simulink model "FormulaElectric"  (R2015a)
settings: Solver=ode1  StartTime=0.0  StopTime=inf  FixedStep=0.001  RelTol=1e-3
InitFcn:
  | %init_dyn_platform
  | FEParameters
StartFcn:
  | tic
StopFcn:
  | toc
undefined symbols (not defined in the file): Battery, Env, magnitude, Motor, RPM2Rad
libraries: vehicleLib x22, mblibv1 x15, driveline x12, fl_lib x8, simulink x6, AMKMotor x4, nesl_utility x4, WheelAssembly x4, ephysenetlib x2, ControllerLib x1, simulink_extras x1
(part 4 of 4)

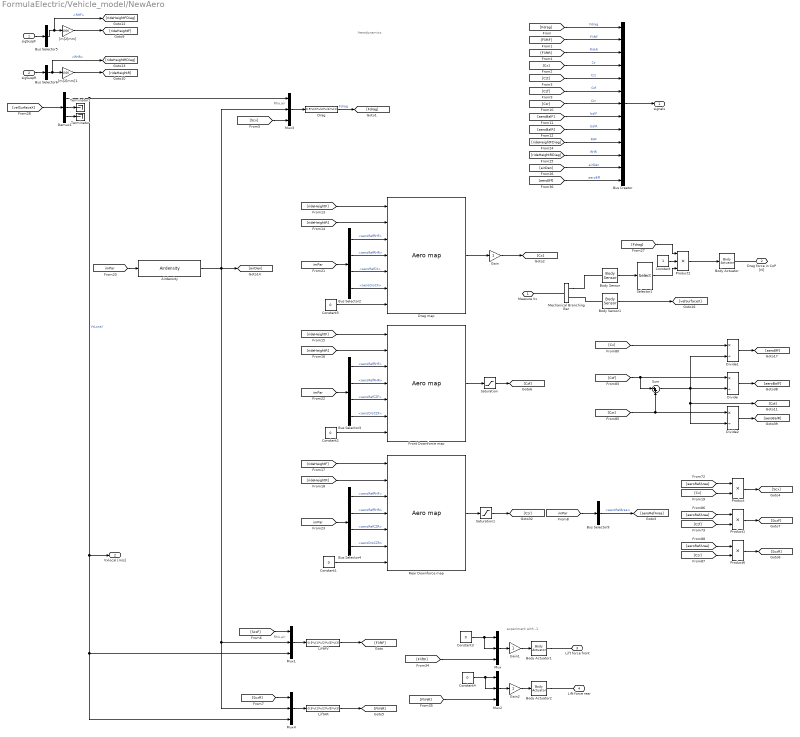
== system FormulaElectric/Vehicle_model/NewAero ==
  note: experiment with -1
  note: Rho,air
  note: Rho,air
  note: Aerodynamics
  sigSuspF : Inport
  sigSuspR : Inport  Port=2
  Airdensity : vehicleLib/Aerodynamics/Aero lib/Airdensity
  Body Actuator : mblibv1/Sensors &  Actuators/Body Actuator  UpdateFromCAD=off  PhysicalDomain=Mechanical  PortType=blob  ActuationStyle=Force  AngleUnits=deg  ArcVelocityUnits=deg/s  ArcAccelerationUnits=deg/s^2  CoordPositionUnits=m  VelocityUnits=m/s  AccelerationUnits=m/s^2  ForceUnits=N  TorqueUnits=N*m  ActiveIO=on  Width=3  DialogClass=MechanicalActuatorBlock  ReferenceFrame=Absolute (World)  Angle=off  CoordPosition=on  Force=on  Torque=off
  Body Actuator1 : mblibv1/Sensors &  Actuators/Body Actuator  UpdateFromCAD=off  PhysicalDomain=Mechanical  PortType=blob  ActuationStyle=Force  AngleUnits=deg  ArcVelocityUnits=deg/s  ArcAccelerationUnits=deg/s^2  CoordPositionUnits=m  VelocityUnits=m/s  AccelerationUnits=m/s^2  ForceUnits=N  TorqueUnits=N*m  ActiveIO=on  Width=3  DialogClass=MechanicalActuatorBlock  ReferenceFrame=Local (Body CS)  Angle=off  CoordPosition=on  Force=on  Torque=off
  Body Actuator2 : mblibv1/Sensors &  Actuators/Body Actuator  UpdateFromCAD=off  PhysicalDomain=Mechanical  PortType=blob  ActuationStyle=Force  AngleUnits=deg  ArcVelocityUnits=deg/s  ArcAccelerationUnits=deg/s^2  CoordPositionUnits=m  VelocityUnits=m/s  AccelerationUnits=m/s^2  ForceUnits=N  TorqueUnits=N*m  ActiveIO=on  Width=3  DialogClass=MechanicalActuatorBlock  ReferenceFrame=Local (Body CS)  Angle=off  CoordPosition=on  Force=on  Torque=off
  Body Sensor : mblibv1/Sensors &  Actuators/Body Sensor  UpdateFromCAD=off  PhysicalDomain=Mechanical  PortType=blob  Muxed=off  Pose=on  Angle=on  AngleUnits=deg  ArcVelocity=off  ArcVelocityUnits=deg/s  ArcAcceleration=off  ArcAccelerationUnits=deg/s^2  CoordPosition=off  CoordPositionUnits=m  Velocity=off  VelocityUnits=m/s  Acceleration=off  AccelerationUnits=m/s^2  Quaternion=on  QuaternionDT=off  QuaternionDDT=off  QuaternionUnits=off  OutputVector=[ 3 ]  ActiveIO=on  Width=9  DialogClass=MechanicalSensorBlock  ReferenceFrame=Absolute (World)
  Body Sensor1 : mblibv1/Sensors &  Actuators/Body Sensor  UpdateFromCAD=off  PhysicalDomain=Mechanical  PortType=blob  Muxed=off  Pose=off  Angle=on  AngleUnits=deg  ArcVelocity=off  ArcVelocityUnits=deg/s  ArcAcceleration=off  ArcAccelerationUnits=deg/s^2  CoordPosition=off  CoordPositionUnits=m  Velocity=on  VelocityUnits=m/s  Acceleration=off  AccelerationUnits=m/s^2  Quaternion=on  QuaternionDT=off  QuaternionDDT=off  QuaternionUnits=off  OutputVector=[ 3 ]  ActiveIO=on  Width=3  DialogClass=MechanicalSensorBlock  ReferenceFrame=Local (Body CS)
  Bus Creator : BusCreator  Inputs=13
  Bus Selector2 : BusSelector  OutputSignals=aeroRefRHF,aeroRefRHR,aeroRefCX,aeroDrsCX
  Bus Selector3 : BusSelector  OutputSignals=aeroRefRHF,aeroRefRHR,aeroRefCZF,aeroDrsCZF
  Bus Selector4 : BusSelector  OutputSignals=aeroRefRHF,aeroRefRHR,aeroRefCZR,aeroDrsCZR
  Bus Selector5 : BusSelector  OutputSignals=sigSuspRH.RHF
  Bus Selector6 : BusSelector  OutputSignals=sigSuspRH.RHR
  Bus Selector9 : BusSelector  OutputSignals=aeroRefArea
  Constant : Constant
  Constant{1..5} (5 alike) : Constant  Value=0
  Demux1 : Demux  Outputs=3
  Divide : Product  Inputs=*/
  Divide1 : Product  Inputs=*/
  Divide2 : Product  Inputs=*/
  Drag : Fcn  Expr=-0.5*u(2)*u(3)*u(1)*u(1)
  Drag map : vehicleLib/Aerodynamics/Aero lib/Aero map  Tag=Aerodynamics: aero map (do not change this tag)  nb=0
  Front Downforce map : vehicleLib/Aerodynamics/Aero lib/Aero map  Tag=Aerodynamics: aero map (do not change this tag)  nb=1
  Gain : Gain
  Gain1 : Gain
  Gain2 : Gain
  LiftAR : Fcn  Expr=-0.5*u(1)*u(2)*u(3)*u(3)
  LiftAV : Fcn  Expr=-0.5*u(1)*u(2)*u(3)*u(3)
  Mechanical Branching Bar : mblibv1/Utilities/Mechanical Branching Bar  LConnTagsString=_newl0  RConnTagsString=SA0|SA1  UpdateFromCAD=off  DialogClass=MechanicalBranchingBarBlock  NumSAPorts=2
  Mux{,1..4} (5 alike) : Mux  Inputs=3
  Product : Product  RndMeth=Zero
  Product1 : Product  RndMeth=Zero
  Product2 : Product  Inputs=3  RndMeth=Zero
  Product6 : Product  RndMeth=Zero
  Rear Downforce map : vehicleLib/Aerodynamics/Aero lib/Aero map  Tag=Aerodynamics: aero map (do not change this tag)  nb=2
  Saturation : Saturate  UpperLimit=0.2  LowerLimit=0
  Saturation1 : Saturate  UpperLimit=0.25  LowerLimit=0
  Selector1 : Selector  InputPortWidth=9  Indices=[1 2 3]
  Sum : Sum  Inputs=|++
  Terminator : Terminator
  Terminator1 : Terminator
  "[m]2[mm]" : Gain  Gain=1000
  "[m]2[mm]1" : Gain  Gain=1000
  Measure Vx : PMIOPort  Port=1  Side=Right
  Drag force in CoP [N] : PMIOPort  Port=2  Side=Left
  Lift force front : PMIOPort  Port=3  Side=Left
  Lift force rear : PMIOPort  Port=4  Side=Left
  signals : Outport
  Vxlocal [m/s] : Outport  Port=2
  wires:
  Constant/1 -> Product2/2
  Selector1/1 -> Product2/3
  Body Sensor/1 -> Selector1/1
  Product6/1 -> [SczR]
  [aeroRefArea] -> Product6/1
  [Czr] -> Product6/2
  Product1/1 -> [SczF]
  [aeroRefArea] -> Product1/1
  [Czf] -> Product1/2
  Product/1 -> [Scx]
  [aeroRefArea] -> Product/1
  [Cx] -> Product/2
  Bus Selector9/1 -> [aeroRefArea]  "<aeroRefArea>"
  [imPar] -> Bus Selector9/1
  Divide2/1 -> [aeroBalR]
  [Czr] -> Divide2/1, Sum/2
  Divide/1 -> [aeroBalF]
  [Czf] -> Divide/1, Sum/1
  Sum/1 -> Divide/2, [Czt], Divide2/2, Divide1/2
  [Cx] -> Divide1/1
  Bus Creator/1 -> signals/1
  [Fdrag] -> Bus Creator/1  "Fdrag"
  [FliftF] -> Bus Creator/2  "FliftF"
  [Cx] -> Bus Creator/4  "Cx"
  [Czt] -> Bus Creator/5  "Czt"
  [FliftR] -> Bus Creator/3  "FliftR"
  [aeroBalF] -> Bus Creator/8  "balF"
  [Czr] -> Bus Creator/7  "Czr"
  [Czf] -> Bus Creator/6  "Czf"
  [aeroBalR] -> Bus Creator/9  "balR"
  [rideHeightFDiag] -> Bus Creator/10  "RHF"
  [rideHeightRDiag] -> Bus Creator/11  "RHR"
  [airDen] -> Bus Creator/12  "airDen"
  [aeroEff] -> Bus Creator/13  "aeroEff"
  [FliftR] -> Mux2/3
  [FliftF] -> Mux/3
  LiftAV/1 -> [FliftF]
  Drag/1 -> [Fdrag]  "Fdrag"
  Mux1/1 -> LiftAV/1
  Mux3/1 -> Drag/1
  Airdensity/1 -> Mux3/2, Mux1/2, Mux4/2, [airDen]
  [Scx] -> Mux3/3
  [SczF] -> Mux1/1
  Mux4/1 -> LiftAR/1
  [SczR] -> Mux4/1
  LiftAR/1 -> [FliftR]
  "[m]2[mm]"/1 -> [rideHeightF]
  "[m]2[mm]1"/1 -> [rideHeightR]
  sigSuspF/1 -> Bus Selector5/1
  Bus Selector5/1 -> "[m]2[mm]"/1, [rideHeightFDiag]  "<RHF>"
  sigSuspR/1 -> Bus Selector6/1
  Bus Selector6/1 -> "[m]2[mm]1"/1, [rideHeightRDiag]  "<RHR>"
  Demux1/3 -> Terminator/1
  Demux1/2 -> Terminator1/1
  Demux1/1 -> Mux3/1, Mux1/3, Mux4/3, Vxlocal [m/s]/1  "VxLocal"
  [velSurfaceX] -> Demux1/1
  Mux/1 -> Gain1/1
  Mux2/1 -> Gain2/1
  Constant3/1 -> Mux/1, Mux/2
  Constant4/1 -> Mux2/1, Mux2/2
  [Fdrag] -> Product2/1
  Product2/1 -> Body Actuator/1
  Body Sensor1/1 -> [velSurfaceX]
  Drag map/1 -> Gain/1
  [rideHeightF] -> Drag map/1
  [imPar] -> Airdensity/1
  Divide1/1 -> [aeroEff]
  Bus Selector2/3 -> Drag map/5  "<aeroRefCX>"
  Bus Selector2/2 -> Drag map/4  "<aeroRefRHR>"
  Bus Selector2/4 -> Drag map/6  "<aeroDrsCX>"
  [imPar] -> Bus Selector2/1
  [rideHeightR] -> Drag map/2
  Bus Selector2/1 -> Drag map/3  "<aeroRefRHF>"
  Constant5/1 -> Drag map/7
  [rideHeightF] -> Front Downforce map/1
  [rideHeightR] -> Front Downforce map/2
  Constant2/1 -> Front Downforce map/7
  [rideHeightF] -> Rear Downforce map/1
  [rideHeightR] -> Rear Downforce map/2
  Constant1/1 -> Rear Downforce map/7
  Bus Selector3/1 -> Front Downforce map/3  "<aeroRefRHF>"
  [imPar] -> Bus Selector3/1
  Bus Selector3/4 -> Front Downforce map/6  "<aeroDrsCZF>"
  Bus Selector3/2 -> Front Downforce map/4  "<aeroRefRHR>"
  Bus Selector3/3 -> Front Downforce map/5  "<aeroRefCZF>"
  Bus Selector4/1 -> Rear Downforce map/3  "<aeroRefRHF>"
  [imPar] -> Bus Selector4/1
  Bus Selector4/4 -> Rear Downforce map/6  "<aeroDrsCZR>"
  Bus Selector4/2 -> Rear Downforce map/4  "<aeroRefRHR>"
  Bus Selector4/3 -> Rear Downforce map/5  "<aeroRefCZR>"
  Front Downforce map/1 -> Saturation/1
  Rear Downforce map/1 -> Saturation1/1
  Gain/1 -> [Cx]
  Saturation/1 -> [Czf]
  Saturation1/1 -> [Czr]
  Gain1/1 -> Body Actuator1/1
  Gain2/1 -> Body Actuator2/1
  connections:
  Body Sensor1/LConn1 -- Mechanical Branching Bar/RConn2
  Mechanical Branching Bar/RConn1 -- Body Sensor/LConn1
  Mechanical Branching Bar/LConn1 -- Measure Vx/RConn1
  Drag force in CoP [N]/RConn1 -- Body Actuator/RConn1
  Body Actuator1/RConn1 -- Lift force front/RConn1
  Body Actuator2/RConn1 -- Lift force rear/RConn1

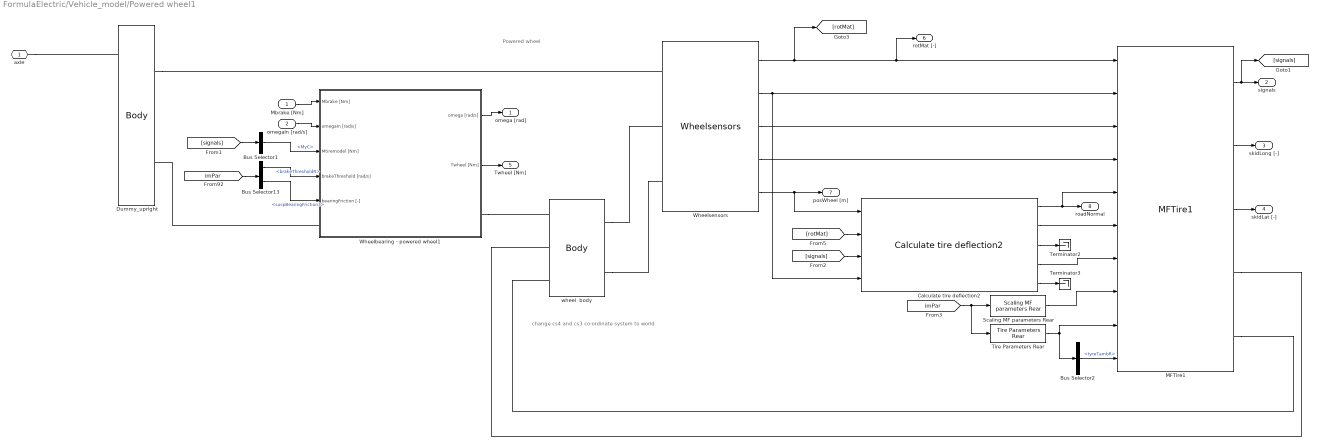
== system FormulaElectric/Vehicle_model/Powered wheel1 ==
  note: change cs4 and cs3 co-ordinate system to world
  note: Powered wheel
  Mbrake [Nm] : Inport
  omegaIn [rad/s] : Inport  Port=2
  Bus Selector1 : BusSelector  OutputSignals=MyC
  Bus Selector13 : BusSelector  OutputSignals=brakeThresholdR,suspBearingFriction3
  Bus Selector2 : BusSelector  OutputSignals=tyreTambR
  Calculate tire deflection2 : vehicleLib/Tire and rim/Tire lib/Calculate tire deflection2
  Dummy_upright : mblibv1/Bodies/Body  LConnTagsString=CS1|CS2|CS5  RConnTagsString=CS9|CS3  UpdateFromCAD=off  DialogClass=MechanicalBodyBlock  Mass=1e-3  MassUnits=kg  InertiaUnits=kg*m^2  Inertia=eye(3)*1e-6  Shape=Cylinder  ShapeDims=[1 1]  ShapeUnits=m  ShapeUse=false  Density=1  DensityUnits=kg/m^3  DensityUse=false  GraphicsMode=MACHINE_DEFAULT  BodyColorSelMode=MACHINE_DEFAULT  BodyColor=[1 0 0]  AttachedToCS=CG  CG=Left$CG$[0 0 0]$CS1$CS1$m$[0 0 0]$Euler X-Y-Z$deg$CS1$false$none  WorkingFrames=Left$CS1$[0 0 0]$Adjoining$Adjoining$m$[0 0 0]$Euler X-Y-Z$deg$Adjoining$true$none#Left$CS2$[suspX tw ahz]$World$World$m$[0 0 0]$Euler X-Y-Z$deg$WORLD$true$none#Right$CS9$[0 0 0]$CS2$CS2$m$[0 0 0]$Euler X-Y-Z$deg$WORLD$true$none#Right$CS3$[0 0 0]$CS1$CS1$m$[0 0 0]$Euler X-Y-Z$deg$CS1$true$none#Left$CS5$[0 0 0]$CS2$CS2$m$[0 0 0]$Euler X-Y-Z$deg$WORLD$true$none  CGPos=[0 0 0]  CGRot=[0 0 0]  CS0Pos=[]  CS0Rot=[]  CS1Pos=[0 0 0]  CS1Rot=[0 0 0]  CS2Pos=[suspX tw ahz]  CS2Rot=[0 0 0]  CS3Pos=[0 0 0]  CS3Rot=[0 0 0]  CS4Pos=[]  CS4Rot=[]  CS5Pos=[0 0 0]  CS5Rot=[0 0 0]  CS6Pos=[]  CS6Rot=[]  CS7Pos=[]  CS7Rot=[]  CS8Pos=[]  CS8Rot=[]  CS9Pos=[0 0 0]  CS9Rot=[0 0 0]  CS10Pos=[]  CS10Rot=[]  CS11Pos=[]  CS11Rot=[]  CS12Pos=[]  CS12Rot=[]  CS13Pos=[]  CS13Rot=[]  CS14Pos=[]  CS14Rot=[]  CS15Pos=[]  CS15Rot=[]  CS16Pos=[]  CS16Rot=[]  CS17Pos=[]  CS17Rot=[]  CS18Pos=[]  CS18Rot=[]  CS19Pos=[]  CS19Rot=[]  CS20Pos=[]  CS20Rot=[]
  MFTire1 : vehicleLib/Tire and rim/Tire lib/MFTire1
  Scaling MF parameters Rear : vehicleLib/Tire and rim/Tire lib/Scaling MF parameters Rear
  Terminator2 : Terminator
  Terminator3 : Terminator
  Tire Parameters Rear : vehicleLib/Tire and rim/Tire lib/Tire Parameters Rear
  Wheelbearing - powered wheel1 : Subsystem  Tag=Tire and rim: wheelbearing powered wheel (do not change this tag)  mask(Wheelbearing powered wheel){}
      mask help:
      | Wheelbearing powered wheel wheel model represents a wheelbearing with stick friction. To be used in combination with the SimMechanics multibody toolbox.
      |
      | Parameters in this model are only used for initialisation during the build process. During simulation with Racer Pro parameters are taken from the car.ini and/or relevant setup.ini.
      |
      | Wheelbearing powered wheel wheel model version: V1.0
      |
      | © Cruden B.V., 2012
  Wheelsensors : vehicleLib/Tire and rim/Tire lib/Wheelsensors
  wheel  body : mblibv1/Bodies/Body  LConnTagsString=CS1|CS2  RConnTagsString=CG|CS4|CS3  UpdateFromCAD=off  DialogClass=MechanicalBodyBlock  Mass=wheelMass  MassUnits=kg  InertiaUnits=kg*m^2  Inertia=inertiaWheel  Shape=Cylinder  ShapeDims=[1 1]  ShapeUnits=m  ShapeUse=false  Density=1  DensityUnits=kg/m^3  DensityUse=false  GraphicsMode=MACHINE_DEFAULT  BodyColorSelMode=MACHINE_DEFAULT  BodyColor=[1 0 0]  AttachedToCS=CG  CG=Right$CG$[0 0 0]$ADJOINING$ADJOINING$m$[0 0 0]$Euler X-Y-Z$deg$ADJOINING$true$none  WorkingFrames=Left$CS1$[0 0 0]$CG$CG$m$[0 0 0]$Euler X-Y-Z$deg$WORLD$true$none#Left$CS2$[0 0 0]$CG$CG$m$[0 0 0]$Euler X-Y-Z$deg$CG$true$none#Right$CS4$[0 0 0]$CG$CG$m$[0 0 0]$Euler X-Y-Z$deg$CG$true$none#Right$CS3$[0 0 0]$CG$CG$m$[0 0 0]$Euler X-Y-Z$deg$CG$true$none  CGPos=[0 0 0]  CGRot=[0 0 0]  CS0Pos=[]  CS0Rot=[]  CS1Pos=[0 0 0]  CS1Rot=[0 0 0]  CS2Pos=[0 0 0]  CS2Rot=[0 0 0]  CS3Pos=[0 0 0]  CS3Rot=[0 0 0]  CS4Pos=[0 0 0]  CS4Rot=[0 0 0]  CS5Pos=[]  CS5Rot=[]  CS6Pos=[]  CS6Rot=[]  CS7Pos=[]  CS7Rot=[]  CS8Pos=[]  CS8Rot=[]  CS9Pos=[]  CS9Rot=[]  CS10Pos=[]  CS10Rot=[]  CS11Pos=[]  CS11Rot=[]  CS12Pos=[]  CS12Rot=[]  CS13Pos=[]  CS13Rot=[]  CS14Pos=[]  CS14Rot=[]  CS15Pos=[]  CS15Rot=[]  CS16Pos=[]  CS16Rot=[]  CS17Pos=[]  CS17Rot=[]  CS18Pos=[]  CS18Rot=[]  CS19Pos=[]  CS19Rot=[]  CS20Pos=[]  CS20Rot=[]
  axle : PMIOPort  Port=1  Side=Left
  omega [rad] : Outport
  signals : Outport  Port=2
  skidLong [-] : Outport  Port=3
  skidLat [-] : Outport  Port=4
  Twheel [Nm] : Outport  Port=5
  rotMat [-] : Outport  Port=6
  posWheel [m] : Outport  Port=7
  roadNormal : Outport  Port=8
  wires:
  Wheelsensors/5 -> Calculate tire deflection2/1, posWheel [m]/1
  Calculate tire deflection2/2 -> MFTire1/6
  Calculate tire deflection2/4 -> MFTire1/7
  Scaling MF parameters Rear/1 -> MFTire1/8
  Bus Selector2/1 -> MFTire1/10  "<tyreTambR>"
  Calculate tire deflection2/5 -> Terminator3/1
  Calculate tire deflection2/3 -> Terminator2/1
  Wheelbearing - powered wheel1/1(omega [rad/s]) -> omega [rad]/1
  Bus Selector13/2 -> Wheelbearing - powered wheel1/5(bearingFriction [-])  "<suspBearingFriction3>"
  Bus Selector13/1 -> Wheelbearing - powered wheel1/4(brakeThreshold [rad/s])  "<brakeThresholdR>"
  [imPar] -> Bus Selector13/1
  Calculate tire deflection2/1 -> MFTire1/5, roadNormal/1
  [signals] -> Calculate tire deflection2/3
  [signals] -> Bus Selector1/1
  Wheelsensors/3 -> MFTire1/3
  Wheelsensors/2 -> Calculate tire deflection2/4, MFTire1/2
  Wheelsensors/1 -> rotMat [-]/1, MFTire1/1, [rotMat]
  MFTire1/1 -> signals/1, [signals]
  Tire Parameters Rear/1 -> MFTire1/9, Bus Selector2/1
  Wheelbearing - powered wheel1/2(Twheel [Nm]) -> Twheel [Nm]/1
  Mbrake [Nm]/1 -> Wheelbearing - powered wheel1/1(Mbrake [Nm])
  omegaIn [rad/s]/1 -> Wheelbearing - powered wheel1/2(omegaIn [rad/s])
  Bus Selector1/1 -> Wheelbearing - powered wheel1/3(Mtiremodel [Nm])  "<MyC>"
  [imPar] -> Scaling MF parameters Rear/1, Tire Parameters Rear/1
  [rotMat] -> Calculate tire deflection2/2
  MFTire1/2 -> skidLong [-]/1
  MFTire1/3 -> skidLat [-]/1
  Wheelsensors/4 -> MFTire1/4
  connections:
  Dummy_upright/RConn1 -- Wheelsensors/LConn1
  axle/RConn1 -- Dummy_upright/LConn1
  wheel  body/LConn1 -- Wheelsensors/LConn2
  wheel  body/LConn2 -- Wheelsensors/LConn3
  Wheelbearing - powered wheel1/RConn1 -- wheel  body/RConn1
  Wheelbearing - powered wheel1/LConn1 -- Dummy_upright/RConn2
  MFTire1/RConn2 -- wheel  body/RConn3
  MFTire1/RConn1 -- wheel  body/RConn2

== system FormulaElectric/Vehicle_model/Subsystem1 ==

== system FormulaElectric/Vehicle_model/World ==
  Custom Joint : mblibv1/Joints/Custom Joint  LConnTagsString=__newl0|SA1  RConnTagsString=__newr0  UpdateFromCAD=off  NumSAPorts=1  CutJoint=off  MarkAsCut=off  Primitives=prismatic  PrimitiveProps=P1$World$[1 0 0]$Prismatic#P2$World$[0 1 0]$Prismatic#P3$World$[0 0 1]$Prismatic#R1$World$[1 0 0]$revolute#R2$World$[0 1 0]$Revolute#R3$World$[0 0 1]$Revolute  DialogClass=JointBlock  R1Axis=[1 0 0]  R2Axis=[0 1 0]  R3Axis=[0 0 1]  P1Axis=[1 0 0]  P2Axis=[0 1 0]  P3Axis=[0 0 1]  SAxis=[]
  Ground : mblibv1/Bodies/Ground  UpdateFromCAD=off  LeftPortType=env  RightPortType=workingframe  PhysicalDomain=Mechanical  DialogClass=GroundBlock  CoordPosition=[0 0 0]  CoordPositionUnits=m  StateVectorMgrId=1  MachineId=[2 0]  ShowEnvPort=on  ParameterChecksum=[1644614091, 3398567388, 4103197596, 3842600041]  TopologyChecksum=[3388181360, 1225848865, 991958222, 3038121235]
  Joint Initial Condition : mblibv1/Sensors &  Actuators/Joint Initial Condition  UpdateFromCAD=off  LeftPortType=blob  RightPortType=blob  PhysicalDomain=mechanical  DialogClass=InitialConditionBlock  InitialConditions=P1$true$81.38$m$deg$0$m/s$deg/s#P2$true$2.75$m$deg$0$m/s$deg/s#P3$true$0$m$deg$0$m/s$deg/s#R1$false$0$m$deg$0$m/s$deg/s#R2$false$0$m$deg$0$m/s$deg/s#R3$false$0$m$deg$0$m/s$deg/s#S$false$0$m$deg$0$m/s$deg/s  P1PIC=81.38  P1VIC=0  P2PIC=2.75  P2VIC=0  P3PIC=0  P3VIC=0  R1PIC=0  R1VIC=0  R2PIC=0  R2VIC=0  R3PIC=0  R3VIC=0  SPIC=0  SVIC=0
  Machine Environment : mblibv1/Bodies/Machine Environment  Tag=Factory ground  PortType=env  PhysicalDomain=Mechanical  DialogTemplateClass=MECH.MachineEnvironment  SyncWhenCopied=off  Gravity=gravityVector  GravityUnits=m/s^2  GravityAsSignal=off  Dimensionality=3D Only  AnalysisType=Forward dynamics  LinearAssemblyTolerance=1e-3  LinearAssemblyToleranceUnits=m  AngularAssemblyTolerance=1e-3  AngularAssemblyToleranceUnits=rad  ConstraintSolverType=Stabilizing  ConstraintRelTolerance=1e-4  ConstraintAbsTolerance=1e-4  UseRobustSingularityHandling=off  RedundancyAnalysisToleranceType=Automatically select tolerance  RedundancyAnalysisTolerance=1e-14  StatePerturbationType=Fixed  PerturbationSize=1e-5  VisualizeMachine=on  BodyVisualizationType=Use model default body geometries  BodyColorSelMode=Use model default  DefaultBodyColor=[1 0 0]
  World : PMIOPort  Port=1  Side=Left
  connections:
  Custom Joint/RConn1 -- World/RConn1
  Custom Joint/LConn2 -- Joint Initial Condition/RConn1
  Machine Environment/RConn1 -- Ground/LConn1
  Custom Joint/LConn1 -- Ground/RConn1

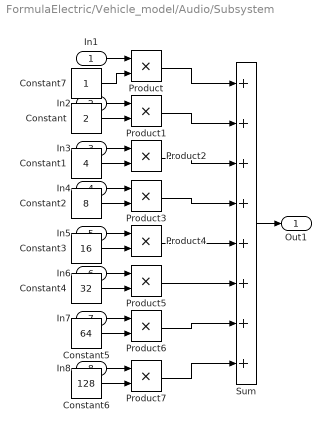
== system FormulaElectric/Vehicle_model/Audio/Subsystem ==
  In1 : Inport
  In2 : Inport  Port=2
  In3 : Inport  Port=3
  In4 : Inport  Port=4
  In5 : Inport  Port=5
  In6 : Inport  Port=6
  In7 : Inport  Port=7
  In8 : Inport  Port=8
  Constant : Constant  Value=2
  Constant1 : Constant  Value=4
  Constant2 : Constant  Value=8
  Constant3 : Constant  Value=16
  Constant4 : Constant  Value=32
  Constant5 : Constant  Value=64
  Constant6 : Constant  Value=128
  Constant7 : Constant
  Product{,1..7} (8 alike) : Product  RndMeth=Zero
  Sum : Sum  Inputs=++++++++
  Out1 : Outport
  wires:
  Constant7/1 -> Product/2
  Constant/1 -> Product1/2
  Constant1/1 -> Product2/2
  Constant2/1 -> Product3/2
  Constant3/1 -> Product4/2
  Constant4/1 -> Product5/2
  Constant5/1 -> Product6/2
  Constant6/1 -> Product7/2
  Product7/1 -> Sum/8
  Product6/1 -> Sum/7
  Product5/1 -> Sum/6
  Product4/1 -> Sum/5
  Product3/1 -> Sum/4
  Product2/1 -> Sum/3
  Product1/1 -> Sum/2
  Product/1 -> Sum/1
  In1/1 -> Product/1
  In2/1 -> Product1/1
  In3/1 -> Product2/1
  In4/1 -> Product3/1
  Sum/1 -> Out1/1
  In5/1 -> Product4/1
  In6/1 -> Product5/1
  In7/1 -> Product6/1
  In8/1 -> Product7/1

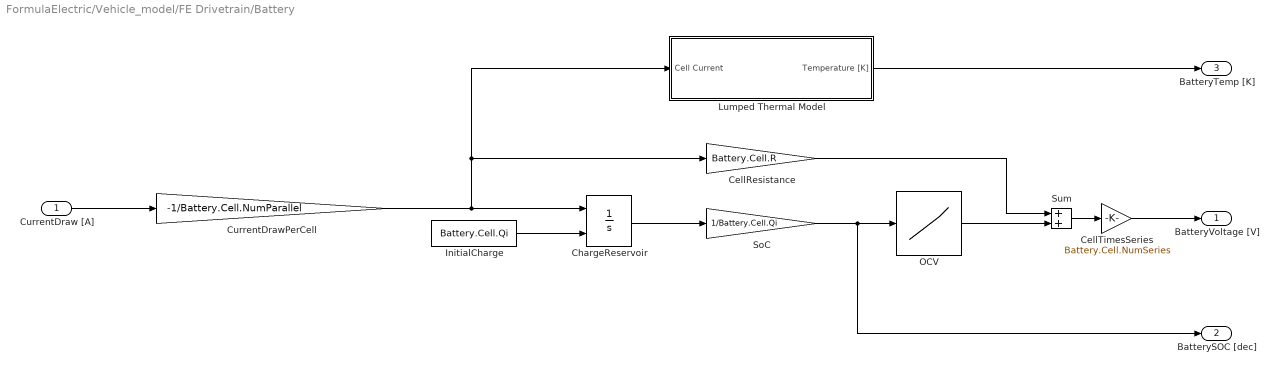
== system FormulaElectric/Vehicle_model/FE Drivetrain/Battery ==
  CurrentDraw [A] : Inport
  CellResistance : Gain  Gain=Battery.Cell.R
  CellTimesSeries : Gain  Gain=Battery.Cell.NumSeries
  ChargeReservoir : Integrator  InitialConditionSource=external
  CurrentDrawPerCell : Gain  Gain=-1/Battery.Cell.NumParallel
  InitialCharge : Constant  Value=Battery.Cell.Qi
  Lumped Thermal Model : Subsystem
  OCV : Lookup_n-D  NumberOfTableDimensions=1  BreakpointsForDimension1=Battery.Cell.VoltOC.SoC  Table=Battery.Cell.VoltOC.Voltage  InternalRulePriority=Speed  RndMeth=Simplest  InputSameDT=on
  SoC : Gain  Gain=1/Battery.Cell.Qi
  Sum : Sum
  BatteryVoltage [V] : Outport
  BatterySOC [dec] : Outport  Port=2
  BatteryTemp [K] : Outport  Port=3
  wires:
  Lumped Thermal Model/1(Temperature [K]) -> BatteryTemp [K]/1
  CurrentDrawPerCell/1 -> ChargeReservoir/1, CellResistance/1, Lumped Thermal Model/1(Cell Current)
  Sum/1 -> CellTimesSeries/1
  OCV/1 -> Sum/2
  CellResistance/1 -> Sum/1
  CellTimesSeries/1 -> BatteryVoltage [V]/1
  SoC/1 -> BatterySOC [dec]/1, OCV/1
  ChargeReservoir/1 -> SoC/1
  InitialCharge/1 -> ChargeReservoir/2
  CurrentDraw [A]/1 -> CurrentDrawPerCell/1

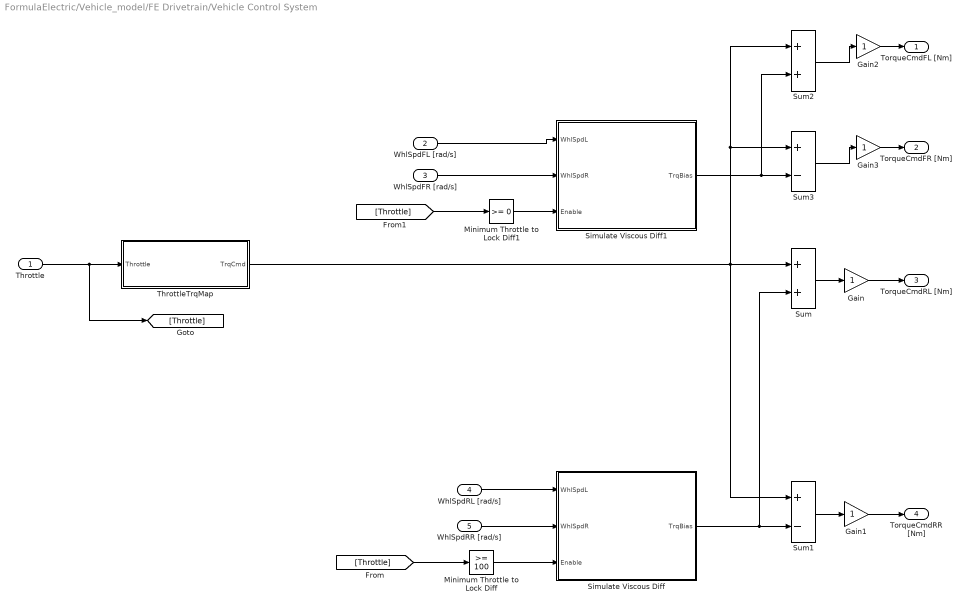
== system FormulaElectric/Vehicle_model/FE Drivetrain/Vehicle Control System ==
  Throttle : Inport
  WhlSpdFL [rad/s] : Inport  Port=2
  WhlSpdFR [rad/s] : Inport  Port=3
  WhlSpdRL [rad/s] : Inport  Port=4
  WhlSpdRR [rad/s] : Inport  Port=5
  Gain{,1..3} (4 alike) : Gain
  Minimum Throttle to Lock Diff : simulink/Logic and Bit Operations/Compare To Constant  relop=>=  const=100  OutDataTypeStr=boolean
  Minimum Throttle to Lock Diff1 : simulink/Logic and Bit Operations/Compare To Constant  relop=>=  const=0  OutDataTypeStr=boolean
  Simulate Viscous Diff : Subsystem
  Simulate Viscous Diff1 : Subsystem
  Sum : Sum
  Sum1 : Sum  Inputs=+-
  Sum2 : Sum
  Sum3 : Sum  Inputs=+-
  ThrottleTrqMap : Subsystem
  TorqueCmdFL [Nm] : Outport
  TorqueCmdFR [Nm] : Outport  Port=2
  TorqueCmdRL [Nm] : Outport  Port=3
  TorqueCmdRR [Nm] : Outport  Port=4
  wires:
  ThrottleTrqMap/1(TrqCmd) -> Sum3/1, Sum2/1, Sum1/1, Sum/1
  WhlSpdRL [rad/s]/1 -> Simulate Viscous Diff/1(WhlSpdL)
  WhlSpdRR [rad/s]/1 -> Simulate Viscous Diff/2(WhlSpdR)
  Simulate Viscous Diff/1(TrqBias) -> Sum1/2, Sum/2
  Sum/1 -> Gain/1
  Sum1/1 -> Gain1/1
  Throttle/1 -> [Throttle], ThrottleTrqMap/1(Throttle)
  [Throttle] -> Minimum Throttle to Lock Diff/1
  Minimum Throttle to Lock Diff/1 -> Simulate Viscous Diff/3(Enable)
  Gain/1 -> TorqueCmdRL [Nm]/1
  Gain1/1 -> TorqueCmdRR [Nm]/1
  WhlSpdFL [rad/s]/1 -> Simulate Viscous Diff1/1(WhlSpdL)
  WhlSpdFR [rad/s]/1 -> Simulate Viscous Diff1/2(WhlSpdR)
  [Throttle] -> Minimum Throttle to Lock Diff1/1
  Minimum Throttle to Lock Diff1/1 -> Simulate Viscous Diff1/3(Enable)
  Simulate Viscous Diff1/1(TrqBias) -> Sum2/2, Sum3/2
  Sum2/1 -> Gain2/1
  Sum3/1 -> Gain3/1
  Gain2/1 -> TorqueCmdFL [Nm]/1
  Gain3/1 -> TorqueCmdFR [Nm]/1

== system FormulaElectric/Vehicle_model/FE Drivetrain/Wheel Assembly ==
  WhlFdbkTrq [Nm] : Inport
  Motion Sensor1 : driveline/Sensors & Actuators/Motion Sensor  Angle=off  x0=0  Velocity=on  Acceleration=off
  Torque Actuator1 : driveline/Sensors & Actuators/Torque Actuator
  driveAxleInertiaR : driveline/Solver & Inertias/Inertia  PortType=p1  BlockClass=Inertia  PhysicalDomain=driveline_domain  I=0.5  Ip=[]  Iv=[]  ShowLeft=on  ShowRight=off
  WhlIn : PMIOPort  Port=1  Side=Left
  WheelSpeed [Rad/s] : Outport
  wires:
  Motion Sensor1/1 -> WheelSpeed [Rad/s]/1  "omegaR"
  WhlFdbkTrq [Nm]/1 -> Torque Actuator1/1
  connections:
  WhlIn/RConn1 -- Motion Sensor1/LConn1 -- Torque Actuator1/RConn1 -- driveAxleInertiaR/LConn1

== system FormulaElectric/Vehicle_model/FE Drivetrain/Wheel Assembly1 ==
  WhlFdbkTrq [Nm] : Inport
  Motion Sensor1 : driveline/Sensors & Actuators/Motion Sensor  Angle=off  x0=0  Velocity=on  Acceleration=off
  Torque Actuator1 : driveline/Sensors & Actuators/Torque Actuator
  driveAxleInertiaR : driveline/Solver & Inertias/Inertia  PortType=p1  BlockClass=Inertia  PhysicalDomain=driveline_domain  I=0.5  Ip=[]  Iv=[]  ShowLeft=on  ShowRight=off
  WhlIn : PMIOPort  Port=1  Side=Left
  WheelSpeed [Rad/s] : Outport
  wires:
  Motion Sensor1/1 -> WheelSpeed [Rad/s]/1  "omegaR"
  WhlFdbkTrq [Nm]/1 -> Torque Actuator1/1
  connections:
  WhlIn/RConn1 -- Motion Sensor1/LConn1 -- Torque Actuator1/RConn1 -- driveAxleInertiaR/LConn1

== system FormulaElectric/Vehicle_model/FE Drivetrain/Wheel Assembly2 ==
  WhlFdbkTrq [Nm] : Inport
  Motion Sensor1 : driveline/Sensors & Actuators/Motion Sensor  Angle=off  x0=0  Velocity=on  Acceleration=off
  Torque Actuator1 : driveline/Sensors & Actuators/Torque Actuator
  driveAxleInertiaR : driveline/Solver & Inertias/Inertia  PortType=p1  BlockClass=Inertia  PhysicalDomain=driveline_domain  I=0.5  Ip=[]  Iv=[]  ShowLeft=on  ShowRight=off
  WhlIn : PMIOPort  Port=1  Side=Left
  WheelSpeed [Rad/s] : Outport
  wires:
  Motion Sensor1/1 -> WheelSpeed [Rad/s]/1  "omegaR"
  WhlFdbkTrq [Nm]/1 -> Torque Actuator1/1
  connections:
  WhlIn/RConn1 -- Motion Sensor1/LConn1 -- Torque Actuator1/RConn1 -- driveAxleInertiaR/LConn1

== system FormulaElectric/Vehicle_model/FE Drivetrain/Wheel Assembly3 ==
  WhlFdbkTrq [Nm] : Inport
  Motion Sensor1 : driveline/Sensors & Actuators/Motion Sensor  Angle=off  x0=0  Velocity=on  Acceleration=off
  Torque Actuator1 : driveline/Sensors & Actuators/Torque Actuator
  driveAxleInertiaR : driveline/Solver & Inertias/Inertia  PortType=p1  BlockClass=Inertia  PhysicalDomain=driveline_domain  I=0.5  Ip=[]  Iv=[]  ShowLeft=on  ShowRight=off
  WhlIn : PMIOPort  Port=1  Side=Left
  WheelSpeed [Rad/s] : Outport
  wires:
  Motion Sensor1/1 -> WheelSpeed [Rad/s]/1  "omegaR"
  WhlFdbkTrq [Nm]/1 -> Torque Actuator1/1
  connections:
  WhlIn/RConn1 -- Motion Sensor1/LConn1 -- Torque Actuator1/RConn1 -- driveAxleInertiaR/LConn1

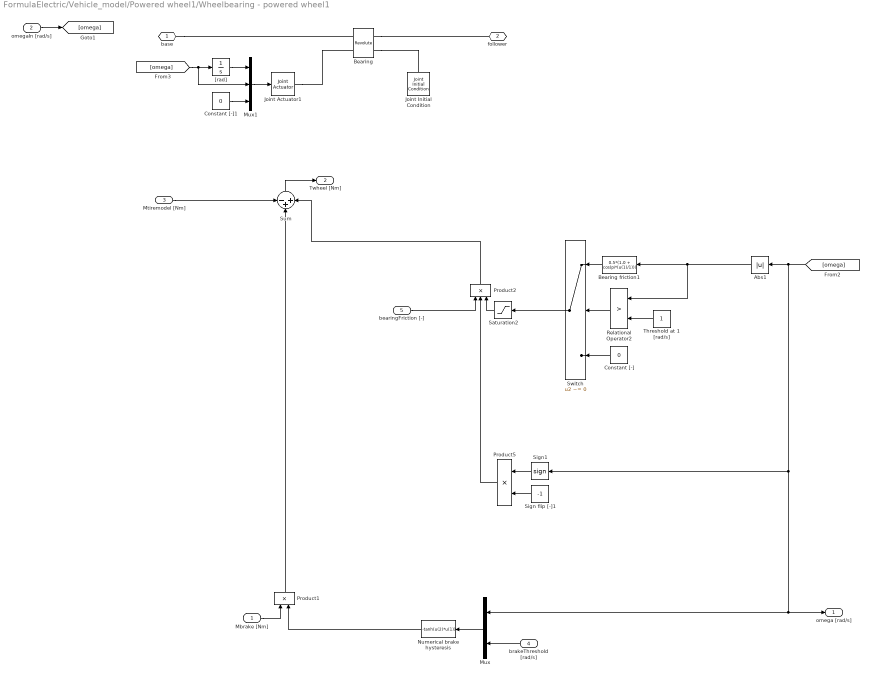
== system FormulaElectric/Vehicle_model/Powered wheel1/Wheelbearing - powered wheel1 ==
  Mbrake [Nm] : Inport
  omegaIn [rad/s] : Inport  Port=2
  Mtiremodel [Nm] : Inport  Port=3
  brakeThreshold [rad/s] : Inport  Port=4
  bearingFriction [-] : Inport  Port=5
  Abs1 : Abs
  Bearing : mblibv1/Joints/Revolute  LConnTagsString=__newl0|SA1  RConnTagsString=__newr0|SA1  UpdateFromCAD=off  NumSAPorts=2  CutJoint=off  MarkAsCut=off  Primitives=revolute  PrimitiveProps=R1$Base$[0 1 0]$revolute  DialogClass=JointBlock  R1Axis=[0 1 0]
  Bearing friction1 : Fcn  Expr=0.5*(1.0 + cos(pi*(u(1)/1)))
  Constant [-] : Constant  Value=0
  Constant [-]1 : Constant  Value=0
  Joint Actuator1 : mblibv1/Sensors &  Actuators/Joint Actuator  UpdateFromCAD=off  PhysicalDomain=Mechanical  PortType=blob  ActuationStyle=Motion  AngleUnits=rad  ArcVelocityUnits=rad/s  ArcAccelerationUnits=rad/s^2  CoordPositionUnits=m  VelocityUnits=m/s  AccelerationUnits=m/s^2  ForceUnits=N  TorqueUnits=N*m  ActiveIO=on  Width=3  DialogClass=MechanicalActuatorBlock  Primitive=R1  ReferenceFrame=Absolute (World)
  Joint Initial Condition : mblibv1/Sensors &  Actuators/Joint Initial Condition  UpdateFromCAD=off  LeftPortType=blob  RightPortType=blob  PhysicalDomain=Mechanical  DialogClass=InitialConditionBlock  InitialConditions=P1$false$0$m$rad$0$m/s$rad/s#P2$false$0$m$rad$0$m/s$rad/s#P3$false$0$m$rad$0$m/s$rad/s#R1$true$0$m$rad$0$m/s$rad/s#R2$false$0$m$rad$Vx/0.284$m/s$rad/s#R3$false$0$m$rad$0$m/s$rad/s#S$false$0$m$rad$0$m/s$rad/s  P1PIC=0  P1VIC=0  P2PIC=0  P2VIC=0  P3PIC=0  P3VIC=0  R1PIC=0  R1VIC=0  R2PIC=0  R2VIC=0  R3PIC=0  R3VIC=0  SPIC=0  SVIC=0
  Mux : Mux  Inputs=2
  Mux1 : Mux  Inputs=3
  Numerical brake hysteresis : Fcn  Expr=-tanh(u(2)*u(1))
  Product1 : Product  SaturateOnIntegerOverflow=on  InputSameDT=on  OutDataTypeStr=Inherit: Same as first input
  Product2 : Product  Inputs=3  SaturateOnIntegerOverflow=on  InputSameDT=on  OutDataTypeStr=Inherit: Same as first input
  Product5 : Product  SaturateOnIntegerOverflow=on  InputSameDT=on  OutDataTypeStr=Inherit: Same as first input
  Relational Operator2 : RelationalOperator  Operator=>  OutDataTypeStr=boolean
  Saturation2 : Saturate  UpperLimit=1  LowerLimit=0
  Sign flip [-]1 : Constant  Value=-1
  Sign1 : Signum
  Sum : Sum  Inputs=-++
  Switch : Switch  Criteria=u2 ~= 0
  Threshold at 1 [rad/s] : Constant
  "[rad]" : Integrator
  base : PMIOPort  Port=1  Side=Left
  follower : PMIOPort  Port=2  Side=Right
  omega [rad/s] : Outport
  Twheel [Nm] : Outport  Port=2
  wires:
  brakeThreshold [rad/s]/1 -> Mux/2
  Product2/1 -> Sum/3
  Sign flip [-]1/1 -> Product5/2
  bearingFriction [-]/1 -> Product2/1
  Switch/1 -> Saturation2/1
  Constant [-]/1 -> Switch/3
  Bearing friction1/1 -> Switch/1
  Relational Operator2/1 -> Switch/2
  Abs1/1 -> Bearing friction1/1, Relational Operator2/1
  Threshold at 1 [rad/s]/1 -> Relational Operator2/2
  [omega] -> Mux/1, omega [rad/s]/1, Sign1/1, Abs1/1
  Saturation2/1 -> Product2/3
  Sign1/1 -> Product5/1
  Product5/1 -> Product2/2
  [omega] -> Mux1/2, "[rad]"/1
  "[rad]"/1 -> Mux1/1
  Mux1/1 -> Joint Actuator1/1
  omegaIn [rad/s]/1 -> [omega]
  Product1/1 -> Sum/2
  Mtiremodel [Nm]/1 -> Sum/1
  Numerical brake hysteresis/1 -> Product1/2
  Mux/1 -> Numerical brake hysteresis/1
  Mbrake [Nm]/1 -> Product1/1
  Sum/1 -> Twheel [Nm]/1
  Constant [-]1/1 -> Mux1/3
  connections:
  Joint Actuator1/RConn1 -- Bearing/LConn2
  Bearing/RConn2 -- Joint Initial Condition/RConn1
  Bearing/RConn1 -- follower/RConn1
  base/RConn1 -- Bearing/LConn1

== system FormulaElectric/Vehicle_model/FE Drivetrain/Battery/Lumped Thermal Model ==
  Cell Current : Inport
  CellResistance1 : Gain  Gain=Battery.Cell.R
  Environment Air : Subsystem
  Heat Source : Subsystem
  Math Function : Math  Operator=magnitude^2  SaturateOnIntegerOverflow=on
  No_Cells : Gain  Gain=Battery.Cell.NumParallel * Battery.Cell.NumSeries
  Solver Configuration : nesl_utility/Solver Configuration  PhysicalDomain=network_engine_domain  SubClassName=solver  LeftPortType=input  RightPortType=generic  Accelerate=off  Tones=[]  Harmonics=[]  SimulateNoise=off  Profile=off  UseLocalSampling=off  EnableSwitchedLinearOptims=on  FrequencyDomain=off  UseCCode=off  RelTol=0.001  AbsTol=1e-06  MinStep=1e-09  ToWorkspace=off  RevertToSquareIcSolve=off  NumHomotopyIterations=100  DoDC=off  ResidualTolerance=1e-09  UseLocalSolver=off  LocalSolverChoice=NE_BACKWARD_EULER_ADVANCER  LocalSolverSampleTime=0.001  DoFixedCost=off  MaxNonlinIter=3  MaxModeIter=2  LinearAlgebra=Sparse  DelaysMemoryBudget=1024  AutomaticFiltering=on  FilteringTimeConstant=0.001
  Temperature Sensor : Subsystem
  Thermal Mass : fl_lib/Thermal/Thermal Elements/Thermal Mass  mass=Battery.m kg  sp_heat=Battery.c J/kg/K  Q_specify=off  Q_priority=High  Q=0 J/s  T_specify=off  T_priority=High  T=300 K
  Temperature [K] : Outport
  wires:
  Cell Current/1 -> Math Function/1
  Temperature Sensor/1(Temperature [K]) -> Temperature [K]/1
  No_Cells/1 -> Heat Source/1(Q)
  CellResistance1/1 -> No_Cells/1
  Math Function/1 -> CellResistance1/1
  connections:
  Thermal Mass/LConn1 -- Solver Configuration/RConn1 -- Heat Source/RConn1 -- Temperature Sensor/LConn1 -- Environment Air/RConn1

== system FormulaElectric/Vehicle_model/FE Drivetrain/Vehicle Control System/Simulate Viscous Diff ==
  note: Add Trq to Left Wheel
  WhlSpdL : Inport
  WhlSpdR : Inport  Port=2
  Enable : Inport  Port=3
  AxleStiffness : Gain  Gain=0.5
  Product : Product
  Subtract : Sum  Inputs=-+
  TrqSplit : Gain  Gain=1/2
  TrqBias : Outport
  wires:
  Subtract/1 -> AxleStiffness/1
  WhlSpdL/1 -> Subtract/1
  WhlSpdR/1 -> Subtract/2
  AxleStiffness/1 -> TrqSplit/1
  Enable/1 -> Product/2
  Product/1 -> TrqBias/1
  TrqSplit/1 -> Product/1

== system FormulaElectric/Vehicle_model/FE Drivetrain/Vehicle Control System/Simulate Viscous Diff1 ==
  note: Add Trq to Left Wheel
  WhlSpdL : Inport
  WhlSpdR : Inport  Port=2
  Enable : Inport  Port=3
  AxleStiffness : Gain  Gain=0.5
  Product : Product
  Subtract : Sum  Inputs=-+
  TrqSplit : Gain  Gain=1/2
  TrqBias : Outport
  wires:
  Subtract/1 -> AxleStiffness/1
  WhlSpdL/1 -> Subtract/1
  WhlSpdR/1 -> Subtract/2
  AxleStiffness/1 -> TrqSplit/1
  Enable/1 -> Product/2
  Product/1 -> TrqBias/1
  TrqSplit/1 -> Product/1

== system FormulaElectric/Vehicle_model/FE Drivetrain/Vehicle Control System/ThrottleTrqMap ==
  Throttle : Inport
  Constant4 : Constant  Value=Motor.PeakTrq
  Product : Product
  TrqCmd : Outport
  wires:
  Product/1 -> TrqCmd/1
  Constant4/1 -> Product/1
  Throttle/1 -> Product/2

== system FormulaElectric/Vehicle_model/FE Drivetrain/Battery/Lumped Thermal Model/Environment Air ==
  Ambient Air : Constant  Value=Env.AmbTemp
  Convective Heat Transfer : fl_lib/Thermal/Thermal Elements/Convective Heat Transfer  area=Battery.SA m^2  heat_tr_coeff=Env.NaturalConvection.K W/(m^2 * K)  Q_specify=off  Q_priority=High  Q=0 J/s  T_specify=off  T_priority=High  T=0 K
  Ideal Temperature Source : fl_lib/Thermal/Thermal Sources/Ideal Temperature Source
  Simulink-PS Converter : nesl_utility/Simulink-PS Converter  PhysicalDomain=network_engine_domain  SubClassName=ps_input  LeftPortType=input  RightPortType=output  PseudoPeriodic=off  Frequencies=[]  NoiseDistribution=none  NoiseParameters=[]  Unit=1  AffineConversion=off  InputFiltering=off  SimscapeFilterOrder=1  InputFilterTimeConstant=0.001  UdotUserProvided=1
  Thermal Reference : fl_lib/Thermal/Thermal Elements/Thermal Reference
  Connection : PMIOPort  Port=1  Side=Right
  wires:
  Ambient Air/1 -> Simulink-PS Converter/1
  connections:
  Convective Heat Transfer/RConn1 -- Connection/RConn1
  Thermal Reference/LConn1 -- Ideal Temperature Source/RConn2
  Simulink-PS Converter/RConn1 -- Ideal Temperature Source/RConn1
  Ideal Temperature Source/LConn1 -- Convective Heat Transfer/LConn1

== system FormulaElectric/Vehicle_model/FE Drivetrain/Battery/Lumped Thermal Model/Heat Source ==
  Q : Inport
  Ideal Heat Flow Source : fl_lib/Thermal/Thermal Sources/Ideal Heat Flow Source
  Simulink-PS Converter : nesl_utility/Simulink-PS Converter  PhysicalDomain=network_engine_domain  SubClassName=ps_input  LeftPortType=input  RightPortType=output  PseudoPeriodic=off  Frequencies=[]  NoiseDistribution=none  NoiseParameters=[]  Unit=1  AffineConversion=off  InputFiltering=off  SimscapeFilterOrder=1  InputFilterTimeConstant=0.001  UdotUserProvided=1
  Thermal Reference : fl_lib/Thermal/Thermal Elements/Thermal Reference
  Connection : PMIOPort  Port=1  Side=Right
  wires:
  Q/1 -> Simulink-PS Converter/1
  connections:
  Ideal Heat Flow Source/LConn1 -- Connection/RConn1
  Thermal Reference/LConn1 -- Ideal Heat Flow Source/RConn2
  Simulink-PS Converter/RConn1 -- Ideal Heat Flow Source/RConn1

== system FormulaElectric/Vehicle_model/FE Drivetrain/Battery/Lumped Thermal Model/Temperature Sensor ==
  Ideal Temperature Sensor : fl_lib/Thermal/Thermal Sensors/Ideal Temperature Sensor
  PS-Simulink Converter : nesl_utility/PS-Simulink Converter  PhysicalDomain=network_engine_domain  SubClassName=ps_output  LeftPortType=input  RightPortType=output  PseudoPeriodic=off  Frequencies=[]  Unit=1  AffineConversion=off
  Thermal Reference : fl_lib/Thermal/Thermal Elements/Thermal Reference
  Connection : PMIOPort  Port=1  Side=Left
  Temperature [K] : Outport
  wires:
  PS-Simulink Converter/1 -> Temperature [K]/1
  connections:
  Ideal Temperature Sensor/RConn1 -- Thermal Reference/LConn1
  PS-Simulink Converter/LConn1 -- Ideal Temperature Sensor/RConn2
  Ideal Temperature Sensor/LConn1 -- Connection/RConn1

== matlab function FormulaElectric/Vehicle_model/MATLAB Function ==
  data: u input; y output
function y = fcn(u)
%#codegen
y = sqrt(u(1)^2 + u(2)^2 + u(3) ^2);
